simulink model "ONE_STEP_BDF"  (R2019b)
settings: Solver=VariableStepAuto  StartTime=0.0  StopTime=10.0  RelTol=1e-3
undefined symbols (not defined in the file): timeStep
settings Model: Creator=simone  LastModifiedBy=simone

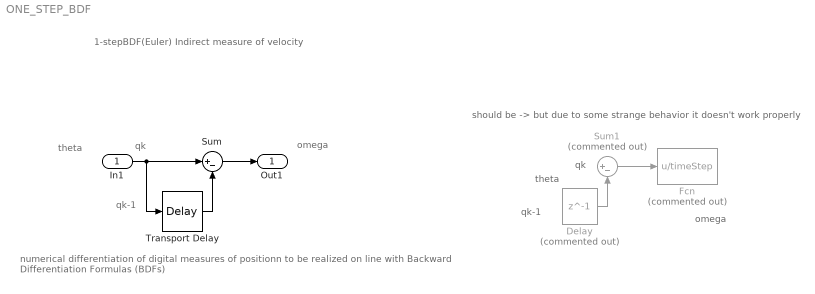
== system ONE_STEP_BDF ==
  note: should be -> but due to some strange behavior it doesn't work properly
  note: theta
  note: omega
  note: qk-1
  note: qk
  note: 1-stepBDF(Euler)
      | Indirect measure of velocity
  note: numerical differentiation of digital measures of positionn to be realized on line with Backward Differentiation Formulas (BDFs)
  note: qk-1
  note: theta
  note: omega
  note: qk
  In1 : Inport
  Delay : Delay  Commented=on  DelayLength=1  InitialCondition=0  SampleTime=timeStep
  Fcn : Fcn  Commented=on  Expr=u/timeStep
  Sum : Sum  Inputs=|+-
  Sum1 : Sum  Commented=on  Inputs=|+-
  Transport Delay : TransportDelay
  Out1 : Outport
  wires:
  Sum/1 -> Out1/1
  In1/1 -> Sum/1, Transport Delay/1
  Transport Delay/1 -> Sum/2
  Sum1/1 -> Fcn/1
  Delay/1 -> Sum1/2
